simulink model "hvac_1zone_v3"  (R2021a)
settings: Solver=ode45  StartTime=0.0  StopTime=Inf  FixedStep=2  RelTol=1e-3  EnableMultiTasking=on
values from neighbouring files (symbols this model uses):
  Ts2 = 600    [main_1zone.m]
undefined symbols (not defined in the file or in its folder): params1, rl
libraries: rllib x1
settings Model: Creator=User  LastModifiedBy=Richi
settings SolverCC: AlgebraicLoopSolver=TrustRegion
settings DataIOCC: LimitDataPoints=on  SaveFormat=Array  SignalLoggingSaveFormat=ModelDataLogs
settings OptimizationCC: LifeSpan=inf
settings DebuggingCC: SolverPrmCheckMsg=warning  MultiTaskDSMMsg=warning  MultiTaskCondExecSysMsg=none  MultiTaskRateTransMsg=warning  AllowSymbolicDim=off  SFUnexpectedBacktrackingDiag=warning  SFNoUnconditionalDefaultTransitionDiag=warning  SFExecutionAtInitializationDiag=none  SFMachineParentedDataDiag=warning  ArithmeticOperatorsInVariantConditions=warning
settings HardwareCC: ProdBitPerPointer=32  ProdBitPerSizeT=32  ProdBitPerPtrDiffT=32  ProdLargestAtomicFloat=None  ProdIntDivRoundTo=Undefined  ProdEndianess=Unspecified  ProdWordSize=32  ProdHWDeviceType=32-bit Generic
settings ModelReferenceCC: PropagateSignalLabelsOutOfModel=off
settings SFSimCC: SimUseLocalCustomCode=off  CustomCodeUndefinedFunction=UseInterfaceOnly
settings RTWCC: RTWUseLocalCustomCode=off
settings CodeAppCC: StateflowObjectComments=on
settings GRTTargetCC: TargetLangStandard=C89/C90 (ANSI)
settings ConfigComp: CovMetricSettings=dw  CovSaveCumulativeToWorkspaceVar=on  CovSaveSingleToWorkspaceVar=on  CovExternalEMLEnable=off

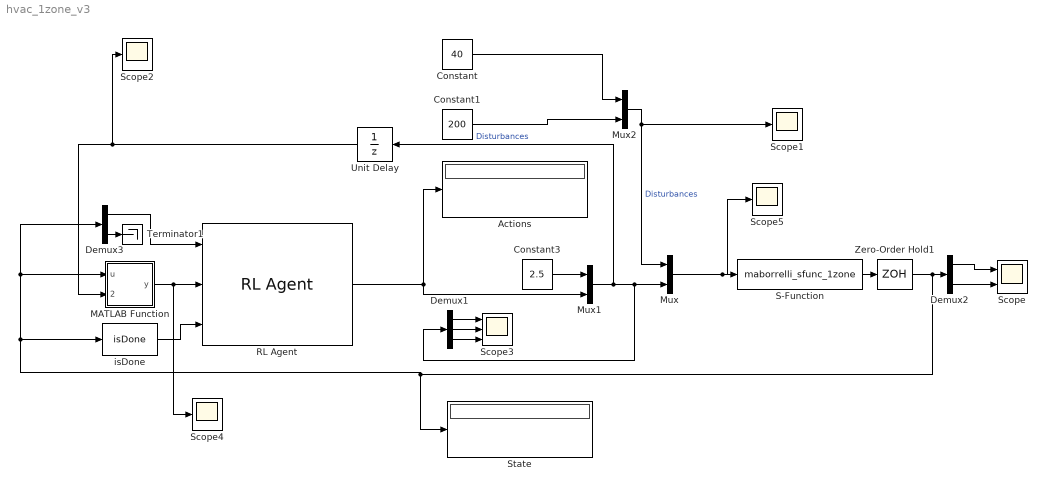
== system hvac_1zone_v3 ==
  Actions : Display
  Constant : Constant  Value=40
  Constant1 : Constant  Value=200
  Constant3 : Constant  Value=2.5
  Demux1 : Demux  Outputs=3
  Demux2 : Demux  Outputs=2
  Demux3 : Demux  Outputs=2
  MATLAB Function : MATLAB Function  TreatAsAtomicUnit=on
  Mux : Mux  Inputs=2
  Mux1 : Mux  Inputs=2
  Mux2 : Mux  Inputs=2
  RL Agent : rllib/RL Agent  Agent=rl.util.PolicyInstance.get('hvac_1zone_v3/RL Agent')  ExternalActionAsInput=off  ProvideCumRwd=off  TreatAsDirectFeedthrough=on
  S-Function : S-Function  FunctionName=maborrelli_sfunc_1zone  Parameters=[34;34],params1  SFunctionDeploymentMode=off  EnableBusSupport=off
  Scope : Scope  NumInputPorts=2
  Scope{1..2,4..5} (4 alike) : Scope
  Scope3 : Scope  NumInputPorts=3
  State : Display
  Terminator1 : Terminator
  Unit Delay : UnitDelay  SampleTime=Ts2  HasFrameUpgradeWarning=on
  Zero-Order Hold1 : ZeroOrderHold  SampleTime=60
  isDone : M-S-Function  FunctionName=isDone
  wires:
  Mux2/1 -> Mux/1, Scope1/1  "Disturbances"
  Constant/1 -> Mux2/1
  RL Agent/1 -> Actions/1, Mux1/2
  isDone/1 -> RL Agent/3
  MATLAB Function/1(y) -> Scope4/1, RL Agent/2
  Constant1/1 -> Mux2/2
  Demux1/2 -> Scope3/2
  Demux1/1 -> Scope3/1
  Demux1/3 -> Scope3/3
  Demux2/1 -> Scope/1
  Demux2/2 -> Scope/2
  Demux3/1 -> RL Agent/1
  Demux3/2 -> Terminator1/1
  Mux1/1 -> Unit Delay/1, Demux1/1, Mux/2  "Disturbances"
  Constant3/1 -> Mux1/1
  Unit Delay/1 -> Scope2/1, MATLAB Function/2(actions)
  Mux/1 -> Scope5/1, S-Function/1
  Zero-Order Hold1/1 -> Demux2/1, MATLAB Function/1(u), Demux3/1, isDone/1, State/1
  S-Function/1 -> Zero-Order Hold1/1

== matlab function hvac_1zone_v3/MATLAB Function ==
  data: u input; y output; actions input
function y = reward(u, actions)
 low = 22;
 high = 25;
 ms = actions(1);
 Dt = actions(2);
 %Añadir energía:
 e = ((-1012/4)*ms*Dt+ 65*(ms)^2)*2.7778e-04;
 reward = -0.8 * e; 
 %disp(length(block.InputPort(1).Data))
 for i=1:1
     %disp(i)
     aux = u(i);
     %disp(aux)
     if (aux < low || aux > high) && (abs(aux - low) >= 1 && abs(aux-high) >= 1)
        %disp(abs(aux - low))
        reward = reward - min( abs(aux - low), abs(aux - high));
        %reward = reward + 0;
        %disp('if13')
     end
     %disp('if1')
     if (aux >= low && aux <= high)
        reward = reward + 0.5;
     end

 end
y = reward;
